simulink model "Part2_linsim"  (R2020b)
settings: Solver=VariableStepAuto  StartTime=0.0  StopTime=66  RelTol=1e-3
undefined symbols (not defined in the file or in its folder): x_star
libraries: cstblocks x6
settings Model: Creator=da_co  LastModifiedBy=da_co

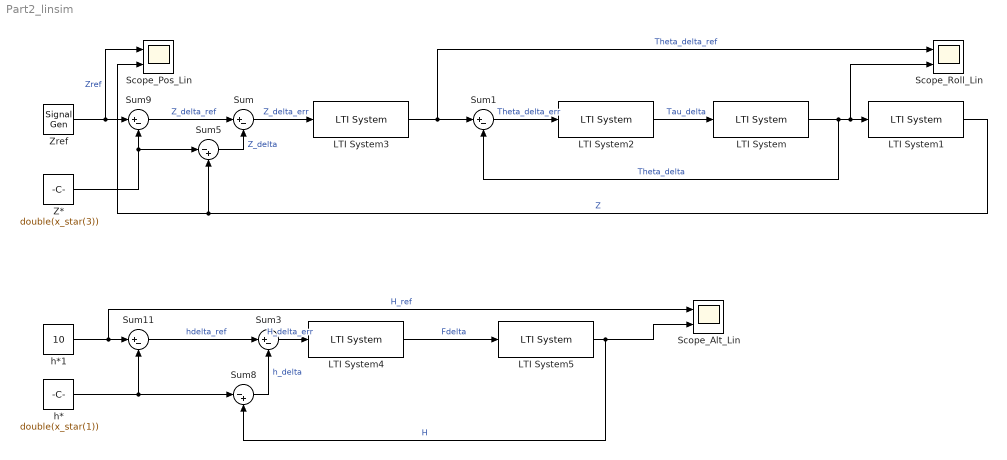
== system Part2_linsim ==
  LTI System : cstblocks/LTI System  sys=G_ThetaTau  IC=[]
  LTI System1 : cstblocks/LTI System  sys=G_ZTheta  IC=[]
  LTI System2 : cstblocks/LTI System  sys=C_roll2  IC=[]
  LTI System3 : cstblocks/LTI System  sys=C_pos2  IC=[]
  LTI System4 : cstblocks/LTI System  sys=C_alt2  IC=[]
  LTI System5 : cstblocks/LTI System  sys=G_HF  IC=[]
  Scope_Alt_Lin : Scope  NumInputPorts=2
  Scope_Pos_Lin : Scope  NumInputPorts=2
  Scope_Roll_Lin : Scope  NumInputPorts=2
  Sum{,1,3,9,11} (5 alike) : Sum  Inputs=|+-
  Sum5 : Sum  Inputs=|-+
  Sum8 : Sum  Inputs=|-+
  Z* : Constant  Value=double(x_star(3))
  Zref : SignalGenerator  WaveForm=square  Amplitude=1.5  Frequency=0.03
  h* : Constant  Value=double(x_star(1))
  h*1 : Constant  Value=10
  wires:
  Zref/1 -> Sum9/1, Scope_Pos_Lin/1  "Zref"
  Sum/1 -> LTI System3/1  "Z_delta_err"
  LTI System3/1 -> Scope_Roll_Lin/1, Sum1/1  "Theta_delta_ref"
  Sum1/1 -> LTI System2/1  "Theta_delta_err"
  LTI System1/1 -> Sum5/2, Scope_Pos_Lin/2  "Z"
  LTI System5/1 -> Sum8/2, Scope_Alt_Lin/2  "H"
  h*1/1 -> Scope_Alt_Lin/1, Sum11/1  "H_ref"
  Z*/1 -> Sum9/2, Sum5/1
  Sum9/1 -> Sum/1  "Z_delta_ref"
  Sum11/1 -> Sum3/1  "hdelta_ref"
  LTI System4/1 -> LTI System5/1  "Fdelta"
  LTI System2/1 -> LTI System/1  "Tau_delta"
  h*/1 -> Sum11/2, Sum8/1
  Sum3/1 -> LTI System4/1  "H_delta_err"
  Sum5/1 -> Sum/2  "Z_delta"
  LTI System/1 -> LTI System1/1, Scope_Roll_Lin/2, Sum1/2  "Theta_delta"
  Sum8/1 -> Sum3/2  "h_delta"
